simulink library "GaitPlayback"  (R2016b)
settings: Solver=VariableStepAuto  StartTime=0.0  StopTime=10.0  RelTol=1e-3
undefined symbols (not defined in the file or in its folder): halfStepStandStartHip, halfStepStandStartKnee, halfStepStopFromStandHip, halfStepStopFromStandKnee, halfStepStopFromSwingHip, halfStepStopFromSwingKnee, halfStepSwingStartHip, halfStepSwingStartKnee, initializeSitDownHip, initializeSitDownKnee, initializeSlopeDownHip, initializeSlopeDownKnee, initializeSlopeUpHip, initializeSlopeUpKnee, initializeSofaDownHip, initializeSofaDownKnee, initializeSofaUpHip, initializeSofaUpKnee, initializeStairsDownHip, initializeStairsDownKnee, initializeStairsUpHip, initializeStairsUpKnee, initializeStandUpHip, initializeStandUpKnee, roughTerrainStepLeftHip, roughTerrainStepLeftKnee, roughTerrainStepRightHip, roughTerrainStepRightKnee, sitDownHip, sitDownKnee, slopeDownLeftHip, slopeDownLeftKnee, slopeDownRightHip, slopeDownRightKnee, slopeUpLeftHip, slopeUpLeftKnee, slopeUpRightHip, slopeUpRightKnee, sofaDownHip, sofaDownKnee, sofaUpHip, sofaUpKnee, stairsDownLeftHip, stairsDownLeftKnee, stairsDownRightHip, stairsDownRightKnee, stairsUpLeftHip, stairsUpLeftKnee, stairsUpRightHip, stairsUpRightKnee, standUpHip, standUpKnee, stepStandLegHip, stepStandLegKnee, stepSwingLegHip, stepSwingLegKnee
libraries: lookUpTotalGaitDynamics x20, GaitPlayback x7, lookUpGaitDynamics x4, VariousLibrary x1
settings Model: Creator=Nathan  LastModifiedBy=MARCH

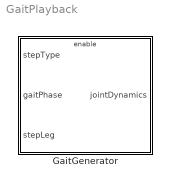
== system GaitPlayback ==
  GaitGenerator : Subsystem

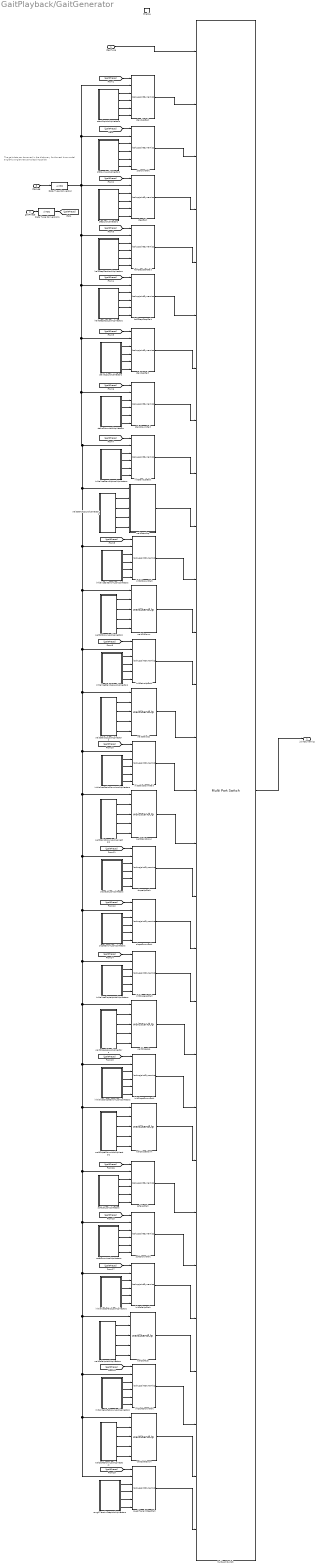
== system GaitPlayback/GaitGenerator ==
  note: The gait data can be saved in the dictionary for the real time model
      | angleHip
      | angleKnee
      | samplepoints/stride
  stepType : Inport
  gaitPhase : Inport  Port=2
  stepLeg : Inport  Port=3
  Enable : EnablePort
  Data Type Conversion : DataTypeConversion  OutDataTypeStr=uint32
  Data Type Conversion1 : DataTypeConversion  OutDataTypeStr=uint32  RndMeth=Nearest
  Multiport Switch : MultiPortSwitch  DataPortOrder=Specify indices  Inputs=4  DataPortIndices={StepType.STANDUP,StepType.SITDOWN,StepType.FULLSTEP,StepType.HALFSTEPSTART,StepType.HALFSTEPSTOP,StepType.STAIRSUPSTEP,StepType.STAIRSDOWNSTEP,StepType.INITIALIZESTANDUP,StepType.WAITSTANDUP,StepType.INITIALIZESITDOWN,StepType.WAITSITDOWN,StepType.INITIALIZESTAIRSUP,StepType.WAITSTAIRSUP,StepType.INITIALIZESTAIRSDOWN,StepType.WAITSTAIRSDOWN,StepType.SLOPEUPSTEP,StepType.SLOPEDOWNSTEP,StepType.INITIALIZESLOPEUP,StepType.WAITSLOPEUP,StepType.INITIALIZESLOPEDOWN,StepType.WAITSLOPEDOWN,StepType.SOFAUPSTEP,StepType.SOFADOWNSTEP,StepType.INITIALIZESOFAUP,StepType.WAITSOFAUP,StepType.INITIALIZESOFADOWN,StepType.WAITSOFADOWN,StepType.ROUGHTERRAINSTEP}  DiagnosticForDefault=None
  halfStepStartGait : lookUpTotalGaitDynamics/lookupJointDynamics
  halfStepStartLookUpVectors : Subsystem
  halfStepStopGait : lookUpTotalGaitDynamics/lookupJointDynamics
  halfStepStopLookUpVectors : Subsystem
  initSitDownGait : lookUpTotalGaitDynamics/lookupJointDynamics
  initSlopeDownGait : lookUpTotalGaitDynamics/lookupJointDynamics
  initSlopeUpGait : lookUpTotalGaitDynamics/lookupJointDynamics
  initSofaDownGait : lookUpTotalGaitDynamics/lookupJointDynamics
  initSofaUpGait : lookUpTotalGaitDynamics/lookupJointDynamics
  initStairsDownGait : lookUpTotalGaitDynamics/lookupJointDynamics
  initStairsUpGait : lookUpTotalGaitDynamics/lookupJointDynamics
  initStandUpGait : lookUpTotalGaitDynamics/lookupJointDynamics
  initializeSitDownLookUpVectors : Subsystem
  initializeSlopeDownLookUpVectors : Subsystem
  initializeSlopeUpLookUpVectors : Subsystem
  initializeSofaDownLookUpVectors : Subsystem
  initializeSofaUpLookUpVectors : Subsystem
  initializeStairsDownLookUpVectors : Subsystem
  initializeStairsUpLookUpVectors : Subsystem
  initializeStandUpLookUpVectors : Subsystem
  roughTerrainStepGait : lookUpTotalGaitDynamics/lookupJointDynamics
  roughTerrainStepLookUpVectors : Subsystem
  sitDownGait : lookUpTotalGaitDynamics/lookupJointDynamics
  sitDownLookUpVectors : Subsystem
  slopeDownGait : lookUpTotalGaitDynamics/lookupJointDynamics
  slopeDownLookUpVectors : Subsystem
  slopeUpGait : lookUpTotalGaitDynamics/lookupJointDynamics
  slopeUpLookUpVectors : Subsystem
  sofaDownGait : lookUpTotalGaitDynamics/lookupJointDynamics
  sofaDownLookUpVectors : Subsystem
  sofaUpGait : lookUpTotalGaitDynamics/lookupJointDynamics
  sofaUpLookUpVectors : Subsystem
  stairsDownGait : lookUpTotalGaitDynamics/lookupJointDynamics
  stairsDownLookUpVectors : Subsystem
  stairsUpGait : lookUpTotalGaitDynamics/lookupJointDynamics
  stairsUpLookUpVectors : Subsystem
  standUpGait : lookUpTotalGaitDynamics/lookupJointDynamics
  standUpLookUpVectors : Subsystem
  stepGait : lookUpTotalGaitDynamics/lookupJointDynamics
  stepLookUpVectors : Subsystem
  waitSitDown : GaitPlayback/GaitGenerator/waitStandUp
  waitSitDownLookUpVectors : Subsystem
  waitSlopeDown : GaitPlayback/GaitGenerator/waitStandUp
  waitSlopeDownLookUpVectors : Subsystem
  waitSlopeUp : GaitPlayback/GaitGenerator/waitStandUp
  waitSlopeUpLookUpVectors : Subsystem
  waitSofaDown : GaitPlayback/GaitGenerator/waitStandUp
  waitSofaDownLookUpVectors : Subsystem
  waitSofaUp : GaitPlayback/GaitGenerator/waitStandUp
  waitSofaUpLookUpVectors : Subsystem
  waitStairsDown : GaitPlayback/GaitGenerator/waitStandUp
  waitStairsDownLookUpVectors : Subsystem
  waitStairsUp : GaitPlayback/GaitGenerator/waitStandUp
  waitStairsUpLookUpVectors : Subsystem
  waitStandUp : Subsystem
  waitStandUpLookUpVectors : Subsystem
  jointDynamics : Outport  OutDataTypeStr=Bus: JointDynamics
  wires:
  stairsUpGait/1 -> Multiport Switch/7
  stairsDownGait/1 -> Multiport Switch/8
  stairsDownLookUpVectors/4(standLegKnee) -> stairsDownGait/6
  stairsDownLookUpVectors/3(standLegHip) -> stairsDownGait/5
  stairsDownLookUpVectors/2(swingLegKnee) -> stairsDownGait/4
  stairsDownLookUpVectors/1(swingLegHip) -> stairsDownGait/3
  [gaitPhase] -> stairsDownGait/1
  stairsUpLookUpVectors/4(standLegKnee) -> stairsUpGait/6
  stairsUpLookUpVectors/3(standLegHip) -> stairsUpGait/5
  stairsUpLookUpVectors/2(swingLegKnee) -> stairsUpGait/4
  stairsUpLookUpVectors/1(swingLegHip) -> stairsUpGait/3
  [gaitPhase] -> stairsUpGait/1
  standUpLookUpVectors/4(standLegKnee) -> standUpGait/6
  standUpLookUpVectors/3(standLegHip) -> standUpGait/5
  standUpLookUpVectors/2(swingLegKnee) -> standUpGait/4
  standUpLookUpVectors/1(swingLegHip) -> standUpGait/3
  gaitPhase/1 -> Data Type Conversion1/1
  Data Type Conversion1/1 -> [gaitPhase]
  [gaitPhase] -> halfStepStopGait/1
  halfStepStopLookUpVectors/4(standLegKnee) -> halfStepStopGait/6
  halfStepStopLookUpVectors/3(standLegHip) -> halfStepStopGait/5
  halfStepStopLookUpVectors/2(swingLegKnee) -> halfStepStopGait/4
  halfStepStopLookUpVectors/1(swingLegHip) -> halfStepStopGait/3
  halfStepStartLookUpVectors/4(standLegKnee) -> halfStepStartGait/6
  halfStepStartLookUpVectors/3(standLegHip) -> halfStepStartGait/5
  halfStepStartLookUpVectors/2(swingLegKnee) -> halfStepStartGait/4
  halfStepStartLookUpVectors/1(swingLegHip) -> halfStepStartGait/3
  sitDownLookUpVectors/1(swingLegHip) -> sitDownGait/3
  sitDownLookUpVectors/2(swingLegKnee) -> sitDownGait/4
  stepLookUpVectors/4(standLegKnee) -> stepGait/6
  [gaitPhase] -> halfStepStartGait/1
  [gaitPhase] -> stepGait/1
  [gaitPhase] -> standUpGait/1
  [gaitPhase] -> sitDownGait/1
  sitDownLookUpVectors/4(standLegKnee) -> sitDownGait/6
  sitDownLookUpVectors/3(standLegHip) -> sitDownGait/5
  stepLookUpVectors/3(standLegHip) -> stepGait/5
  stepLookUpVectors/2(swingLegKnee) -> stepGait/4
  stepLookUpVectors/1(swingLegHip) -> stepGait/3
  halfStepStopGait/1 -> Multiport Switch/6
  halfStepStartGait/1 -> Multiport Switch/5
  stepGait/1 -> Multiport Switch/4
  Multiport Switch/1 -> jointDynamics/1
  standUpGait/1 -> Multiport Switch/2
  stepType/1 -> Multiport Switch/1
  sitDownGait/1 -> Multiport Switch/3
  stepLeg/1 -> Data Type Conversion/1
  initStandUpGait/1 -> Multiport Switch/9
  initializeStandUpLookUpVectors/3(standLegHip) -> initStandUpGait/5
  initializeStandUpLookUpVectors/2(swingLegKnee) -> initStandUpGait/4
  initializeStandUpLookUpVectors/1(swingLegHip) -> initStandUpGait/3
  [gaitPhase] -> initStandUpGait/1
  initializeStandUpLookUpVectors/4(standLegKnee) -> initStandUpGait/6
  waitStandUpLookUpVectors/3(standLegHip) -> waitStandUp/4(standLegHip)
  waitStandUpLookUpVectors/2(swingLegKnee) -> waitStandUp/3(swingLegKnee)
  waitStandUpLookUpVectors/1(swingLegHip) -> waitStandUp/2(swingLegHip)
  waitStandUp/1(jointDynamics1) -> Multiport Switch/10
  waitStandUpLookUpVectors/4(standLegKnee) -> waitStandUp/5(standLegKnee)
  waitSitDownLookUpVectors/3(standLegHip) -> waitSitDown/4
  waitSitDownLookUpVectors/2(swingLegKnee) -> waitSitDown/3
  waitSitDownLookUpVectors/1(swingLegHip) -> waitSitDown/2
  waitSitDown/1 -> Multiport Switch/12
  waitSitDownLookUpVectors/4(standLegKnee) -> waitSitDown/5
  initSitDownGait/1 -> Multiport Switch/11
  initializeSitDownLookUpVectors/3(standLegHip) -> initSitDownGait/5
  initializeSitDownLookUpVectors/2(swingLegKnee) -> initSitDownGait/4
  initializeSitDownLookUpVectors/1(swingLegHip) -> initSitDownGait/3
  [gaitPhase] -> initSitDownGait/1
  initializeSitDownLookUpVectors/4(standLegKnee) -> initSitDownGait/6
  waitStairsUpLookUpVectors/3(standLegHip) -> waitStairsUp/4
  waitStairsUpLookUpVectors/2(swingLegKnee) -> waitStairsUp/3
  waitStairsUpLookUpVectors/1(swingLegHip) -> waitStairsUp/2
  waitStairsUpLookUpVectors/4(standLegKnee) -> waitStairsUp/5
  initializeStairsUpLookUpVectors/3(standLegHip) -> initStairsUpGait/5
  initializeStairsUpLookUpVectors/4(standLegKnee) -> initStairsUpGait/6
  initializeStairsUpLookUpVectors/2(swingLegKnee) -> initStairsUpGait/4
  initializeStairsUpLookUpVectors/1(swingLegHip) -> initStairsUpGait/3
  [gaitPhase] -> initStairsUpGait/1
  waitStairsDownLookUpVectors/3(standLegHip) -> waitStairsDown/4
  waitStairsDownLookUpVectors/2(swingLegKnee) -> waitStairsDown/3
  waitStairsDownLookUpVectors/1(swingLegHip) -> waitStairsDown/2
  waitStairsDownLookUpVectors/4(standLegKnee) -> waitStairsDown/5
  initializeStairsDownLookUpVectors/3(standLegHip) -> initStairsDownGait/5
  initializeStairsDownLookUpVectors/4(standLegKnee) -> initStairsDownGait/6
  initializeStairsDownLookUpVectors/2(swingLegKnee) -> initStairsDownGait/4
  initializeStairsDownLookUpVectors/1(swingLegHip) -> initStairsDownGait/3
  [gaitPhase] -> initStairsDownGait/1
  waitStairsDown/1 -> Multiport Switch/16
  initStairsDownGait/1 -> Multiport Switch/15
  waitStairsUp/1 -> Multiport Switch/14
  initStairsUpGait/1 -> Multiport Switch/13
  slopeUpGait/1 -> Multiport Switch/17
  slopeDownGait/1 -> Multiport Switch/18
  slopeDownLookUpVectors/4(standLegKnee) -> slopeDownGait/6
  slopeDownLookUpVectors/3(standLegHip) -> slopeDownGait/5
  slopeDownLookUpVectors/2(swingLegKnee) -> slopeDownGait/4
  slopeDownLookUpVectors/1(swingLegHip) -> slopeDownGait/3
  [gaitPhase] -> slopeDownGait/1
  slopeUpLookUpVectors/4(standLegKnee) -> slopeUpGait/6
  slopeUpLookUpVectors/3(standLegHip) -> slopeUpGait/5
  slopeUpLookUpVectors/2(swingLegKnee) -> slopeUpGait/4
  slopeUpLookUpVectors/1(swingLegHip) -> slopeUpGait/3
  [gaitPhase] -> slopeUpGait/1
  waitSlopeUpLookUpVectors/3(standLegHip) -> waitSlopeUp/4
  waitSlopeUpLookUpVectors/2(swingLegKnee) -> waitSlopeUp/3
  waitSlopeUpLookUpVectors/1(swingLegHip) -> waitSlopeUp/2
  waitSlopeUpLookUpVectors/4(standLegKnee) -> waitSlopeUp/5
  initializeSlopeUpLookUpVectors/3(standLegHip) -> initSlopeUpGait/5
  initializeSlopeUpLookUpVectors/4(standLegKnee) -> initSlopeUpGait/6
  initializeSlopeUpLookUpVectors/2(swingLegKnee) -> initSlopeUpGait/4
  initializeSlopeUpLookUpVectors/1(swingLegHip) -> initSlopeUpGait/3
  [gaitPhase] -> initSlopeUpGait/1
  waitSlopeDownLookUpVectors/3(standLegHip) -> waitSlopeDown/4
  waitSlopeDownLookUpVectors/2(swingLegKnee) -> waitSlopeDown/3
  waitSlopeDownLookUpVectors/1(swingLegHip) -> waitSlopeDown/2
  waitSlopeDownLookUpVectors/4(standLegKnee) -> waitSlopeDown/5
  initializeSlopeDownLookUpVectors/3(standLegHip) -> initSlopeDownGait/5
  initializeSlopeDownLookUpVectors/4(standLegKnee) -> initSlopeDownGait/6
  initializeSlopeDownLookUpVectors/2(swingLegKnee) -> initSlopeDownGait/4
  initializeSlopeDownLookUpVectors/1(swingLegHip) -> initSlopeDownGait/3
  [gaitPhase] -> initSlopeDownGait/1
  waitSlopeDown/1 -> Multiport Switch/22
  initSlopeDownGait/1 -> Multiport Switch/21
  waitSlopeUp/1 -> Multiport Switch/20
  initSlopeUpGait/1 -> Multiport Switch/19
  sofaUpLookUpVectors/4(standLegKnee) -> sofaUpGait/6
  sofaUpLookUpVectors/3(standLegHip) -> sofaUpGait/5
  sofaUpLookUpVectors/2(swingLegKnee) -> sofaUpGait/4
  sofaUpLookUpVectors/1(swingLegHip) -> sofaUpGait/3
  sofaDownLookUpVectors/1(swingLegHip) -> sofaDownGait/3
  [gaitPhase] -> sofaUpGait/1
  [gaitPhase] -> sofaDownGait/1
  sofaUpGait/1 -> Multiport Switch/23
  sofaDownGait/1 -> Multiport Switch/24
  initSofaUpGait/1 -> Multiport Switch/25
  initializeSofaUpLookUpVectors/3(standLegHip) -> initSofaUpGait/5
  initializeSofaUpLookUpVectors/2(swingLegKnee) -> initSofaUpGait/4
  initializeSofaUpLookUpVectors/1(swingLegHip) -> initSofaUpGait/3
  [gaitPhase] -> initSofaUpGait/1
  initializeSofaUpLookUpVectors/4(standLegKnee) -> initSofaUpGait/6
  waitSofaUpLookUpVectors/3(standLegHip) -> waitSofaUp/4
  waitSofaUpLookUpVectors/2(swingLegKnee) -> waitSofaUp/3
  waitSofaUpLookUpVectors/1(swingLegHip) -> waitSofaUp/2
  waitSofaUp/1 -> Multiport Switch/26
  waitSofaUpLookUpVectors/4(standLegKnee) -> waitSofaUp/5
  waitSofaDownLookUpVectors/3(standLegHip) -> waitSofaDown/4
  waitSofaDownLookUpVectors/2(swingLegKnee) -> waitSofaDown/3
  waitSofaDownLookUpVectors/1(swingLegHip) -> waitSofaDown/2
  waitSofaDown/1 -> Multiport Switch/28
  waitSofaDownLookUpVectors/4(standLegKnee) -> waitSofaDown/5
  initSofaDownGait/1 -> Multiport Switch/27
  initializeSofaDownLookUpVectors/3(standLegHip) -> initSofaDownGait/5
  initializeSofaDownLookUpVectors/2(swingLegKnee) -> initSofaDownGait/4
  initializeSofaDownLookUpVectors/1(swingLegHip) -> initSofaDownGait/3
  [gaitPhase] -> initSofaDownGait/1
  initializeSofaDownLookUpVectors/4(standLegKnee) -> initSofaDownGait/6
  sofaDownLookUpVectors/2(swingLegKnee) -> sofaDownGait/4
  sofaDownLookUpVectors/3(standLegHip) -> sofaDownGait/5
  sofaDownLookUpVectors/4(standLegKnee) -> sofaDownGait/6
  roughTerrainStepLookUpVectors/4(standLegKnee) -> roughTerrainStepGait/6
  roughTerrainStepLookUpVectors/3(standLegHip) -> roughTerrainStepGait/5
  roughTerrainStepLookUpVectors/2(swingLegKnee) -> roughTerrainStepGait/4
  roughTerrainStepLookUpVectors/1(swingLegHip) -> roughTerrainStepGait/3
  [gaitPhase] -> roughTerrainStepGait/1
  roughTerrainStepGait/1 -> Multiport Switch/29
  Data Type Conversion/1 -> standUpGait/2, sitDownGait/2, stairsDownGait/2, initSitDownGait/2, initStairsDownGait/2, initSlopeUpGait/2, waitSlopeUp/1, initSlopeDownGait/2, roughTerrainStepGait/2, waitSofaDown/1, initSofaDownGait/2, waitSofaUp/1, initSofaUpGait/2, sofaDownGait/2, sofaUpGait/2, waitSlopeDown/1, slopeDownGait/2, slopeUpGait/2, waitStairsDown/1, waitStairsUp/1, initStairsUpGait/2, waitSitDown/1, waitStandUp/1(stepLeg), initStandUpGait/2, stairsUpGait/2, halfStepStopGait/2, halfStepStartGait/2, stepGait/2

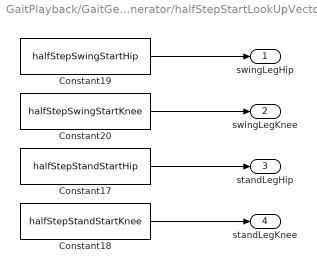
== system GaitPlayback/GaitGenerator/halfStepStartLookUpVectors ==
  Constant17 : Constant  Value=halfStepStandStartHip
  Constant18 : Constant  Value=halfStepStandStartKnee
  Constant19 : Constant  Value=halfStepSwingStartHip
  Constant20 : Constant  Value=halfStepSwingStartKnee
  swingLegHip : Outport
  swingLegKnee : Outport  Port=2
  standLegHip : Outport  Port=3
  standLegKnee : Outport  Port=4
  wires:
  Constant18/1 -> standLegKnee/1
  Constant17/1 -> standLegHip/1
  Constant19/1 -> swingLegHip/1
  Constant20/1 -> swingLegKnee/1

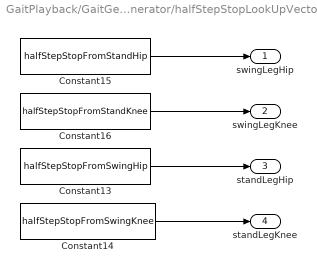
== system GaitPlayback/GaitGenerator/halfStepStopLookUpVectors ==
  Constant13 : Constant  Value=halfStepStopFromSwingHip
  Constant14 : Constant  Value=halfStepStopFromSwingKnee
  Constant15 : Constant  Value=halfStepStopFromStandHip
  Constant16 : Constant  Value=halfStepStopFromStandKnee
  swingLegHip : Outport
  swingLegKnee : Outport  Port=2
  standLegHip : Outport  Port=3
  standLegKnee : Outport  Port=4
  wires:
  Constant14/1 -> standLegKnee/1
  Constant13/1 -> standLegHip/1
  Constant15/1 -> swingLegHip/1
  Constant16/1 -> swingLegKnee/1

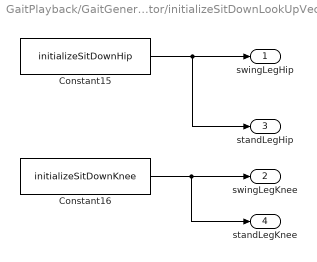
== system GaitPlayback/GaitGenerator/initializeSitDownLookUpVectors ==
  Constant15 : Constant  Value=initializeSitDownHip
  Constant16 : Constant  Value=initializeSitDownKnee
  swingLegHip : Outport
  swingLegKnee : Outport  Port=2
  standLegHip : Outport  Port=3
  standLegKnee : Outport  Port=4
  wires:
  Constant16/1 -> standLegKnee/1, swingLegKnee/1
  Constant15/1 -> standLegHip/1, swingLegHip/1

== system GaitPlayback/GaitGenerator/initializeSlopeDownLookUpVectors ==
  Constant15 : Constant  Value=initializeSlopeDownHip
  Constant16 : Constant  Value=initializeSlopeDownKnee
  swingLegHip : Outport
  swingLegKnee : Outport  Port=2
  standLegHip : Outport  Port=3
  standLegKnee : Outport  Port=4
  wires:
  Constant16/1 -> standLegKnee/1, swingLegKnee/1
  Constant15/1 -> standLegHip/1, swingLegHip/1

== system GaitPlayback/GaitGenerator/initializeSlopeUpLookUpVectors ==
  Constant15 : Constant  Value=initializeSlopeUpHip
  Constant16 : Constant  Value=initializeSlopeUpKnee
  swingLegHip : Outport
  swingLegKnee : Outport  Port=2
  standLegHip : Outport  Port=3
  standLegKnee : Outport  Port=4
  wires:
  Constant16/1 -> standLegKnee/1, swingLegKnee/1
  Constant15/1 -> standLegHip/1, swingLegHip/1

== system GaitPlayback/GaitGenerator/initializeSofaDownLookUpVectors ==
  Constant15 : Constant  Value=initializeSofaDownHip
  Constant16 : Constant  Value=initializeSofaDownKnee
  swingLegHip : Outport
  swingLegKnee : Outport  Port=2
  standLegHip : Outport  Port=3
  standLegKnee : Outport  Port=4
  wires:
  Constant16/1 -> standLegKnee/1, swingLegKnee/1
  Constant15/1 -> standLegHip/1, swingLegHip/1

== system GaitPlayback/GaitGenerator/initializeSofaUpLookUpVectors ==
  Constant15 : Constant  Value=initializeSofaUpHip
  Constant16 : Constant  Value=initializeSofaUpKnee
  swingLegHip : Outport
  swingLegKnee : Outport  Port=2
  standLegHip : Outport  Port=3
  standLegKnee : Outport  Port=4
  wires:
  Constant16/1 -> standLegKnee/1, swingLegKnee/1
  Constant15/1 -> standLegHip/1, swingLegHip/1

== system GaitPlayback/GaitGenerator/initializeStairsDownLookUpVectors ==
  Constant15 : Constant  Value=initializeStairsDownHip
  Constant16 : Constant  Value=initializeStairsDownKnee
  swingLegHip : Outport
  swingLegKnee : Outport  Port=2
  standLegHip : Outport  Port=3
  standLegKnee : Outport  Port=4
  wires:
  Constant16/1 -> standLegKnee/1, swingLegKnee/1
  Constant15/1 -> standLegHip/1, swingLegHip/1

== system GaitPlayback/GaitGenerator/initializeStairsUpLookUpVectors ==
  Constant15 : Constant  Value=initializeStairsUpHip
  Constant16 : Constant  Value=initializeStairsUpKnee
  swingLegHip : Outport
  swingLegKnee : Outport  Port=2
  standLegHip : Outport  Port=3
  standLegKnee : Outport  Port=4
  wires:
  Constant16/1 -> standLegKnee/1, swingLegKnee/1
  Constant15/1 -> standLegHip/1, swingLegHip/1

== system GaitPlayback/GaitGenerator/initializeStandUpLookUpVectors ==
  Constant15 : Constant  Value=initializeStandUpHip
  Constant16 : Constant  Value=initializeStandUpKnee
  swingLegHip : Outport
  swingLegKnee : Outport  Port=2
  standLegHip : Outport  Port=3
  standLegKnee : Outport  Port=4
  wires:
  Constant16/1 -> standLegKnee/1, swingLegKnee/1
  Constant15/1 -> standLegHip/1, swingLegHip/1

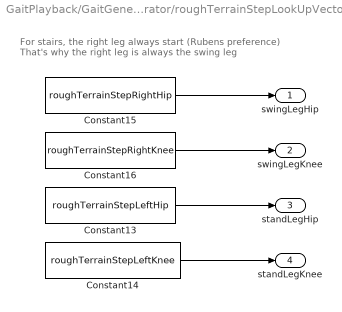
== system GaitPlayback/GaitGenerator/roughTerrainStepLookUpVectors ==
  note: For stairs, the right leg always start (Rubens preference)
      | That's why the right leg is always the swing leg
  Constant13 : Constant  Value=roughTerrainStepLeftHip
  Constant14 : Constant  Value=roughTerrainStepLeftKnee
  Constant15 : Constant  Value=roughTerrainStepRightHip
  Constant16 : Constant  Value=roughTerrainStepRightKnee
  swingLegHip : Outport
  swingLegKnee : Outport  Port=2
  standLegHip : Outport  Port=3
  standLegKnee : Outport  Port=4
  wires:
  Constant14/1 -> standLegKnee/1
  Constant13/1 -> standLegHip/1
  Constant15/1 -> swingLegHip/1
  Constant16/1 -> swingLegKnee/1

== system GaitPlayback/GaitGenerator/sitDownLookUpVectors ==
  Constant12 : Constant  Value=sitDownHip
  Constant7 : Constant  Value=sitDownKnee
  swingLegHip : Outport
  swingLegKnee : Outport  Port=2
  standLegHip : Outport  Port=3
  standLegKnee : Outport  Port=4
  wires:
  Constant12/1 -> swingLegHip/1, standLegHip/1
  Constant7/1 -> swingLegKnee/1, standLegKnee/1

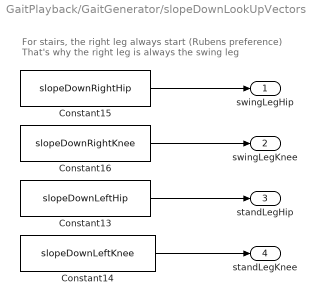
== system GaitPlayback/GaitGenerator/slopeDownLookUpVectors ==
  note: For stairs, the right leg always start (Rubens preference)
      | That's why the right leg is always the swing leg
  Constant13 : Constant  Value=slopeDownLeftHip
  Constant14 : Constant  Value=slopeDownLeftKnee
  Constant15 : Constant  Value=slopeDownRightHip
  Constant16 : Constant  Value=slopeDownRightKnee
  swingLegHip : Outport
  swingLegKnee : Outport  Port=2
  standLegHip : Outport  Port=3
  standLegKnee : Outport  Port=4
  wires:
  Constant14/1 -> standLegKnee/1
  Constant13/1 -> standLegHip/1
  Constant15/1 -> swingLegHip/1
  Constant16/1 -> swingLegKnee/1

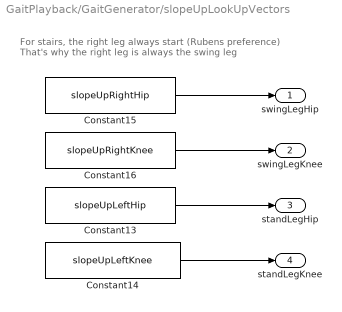
== system GaitPlayback/GaitGenerator/slopeUpLookUpVectors ==
  note: For stairs, the right leg always start (Rubens preference)
      | That's why the right leg is always the swing leg
  Constant13 : Constant  Value=slopeUpLeftHip
  Constant14 : Constant  Value=slopeUpLeftKnee
  Constant15 : Constant  Value=slopeUpRightHip
  Constant16 : Constant  Value=slopeUpRightKnee
  swingLegHip : Outport
  swingLegKnee : Outport  Port=2
  standLegHip : Outport  Port=3
  standLegKnee : Outport  Port=4
  wires:
  Constant14/1 -> standLegKnee/1
  Constant13/1 -> standLegHip/1
  Constant15/1 -> swingLegHip/1
  Constant16/1 -> swingLegKnee/1

== system GaitPlayback/GaitGenerator/sofaDownLookUpVectors ==
  Constant12 : Constant  Value=sofaDownHip
  Constant7 : Constant  Value=sofaDownKnee
  swingLegHip : Outport
  swingLegKnee : Outport  Port=2
  standLegHip : Outport  Port=3
  standLegKnee : Outport  Port=4
  wires:
  Constant12/1 -> swingLegHip/1, standLegHip/1
  Constant7/1 -> swingLegKnee/1, standLegKnee/1

== system GaitPlayback/GaitGenerator/sofaUpLookUpVectors ==
  standUpHip : Constant  Value=sofaUpHip
  standUpKnee : Constant  Value=sofaUpKnee
  swingLegHip : Outport
  swingLegKnee : Outport  Port=2
  standLegHip : Outport  Port=3
  standLegKnee : Outport  Port=4
  wires:
  standUpHip/1 -> swingLegHip/1, standLegHip/1
  standUpKnee/1 -> swingLegKnee/1, standLegKnee/1

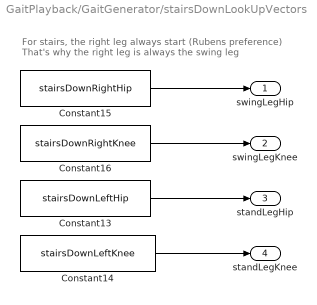
== system GaitPlayback/GaitGenerator/stairsDownLookUpVectors ==
  note: For stairs, the right leg always start (Rubens preference)
      | That's why the right leg is always the swing leg
  Constant13 : Constant  Value=stairsDownLeftHip
  Constant14 : Constant  Value=stairsDownLeftKnee
  Constant15 : Constant  Value=stairsDownRightHip
  Constant16 : Constant  Value=stairsDownRightKnee
  swingLegHip : Outport
  swingLegKnee : Outport  Port=2
  standLegHip : Outport  Port=3
  standLegKnee : Outport  Port=4
  wires:
  Constant14/1 -> standLegKnee/1
  Constant13/1 -> standLegHip/1
  Constant15/1 -> swingLegHip/1
  Constant16/1 -> swingLegKnee/1

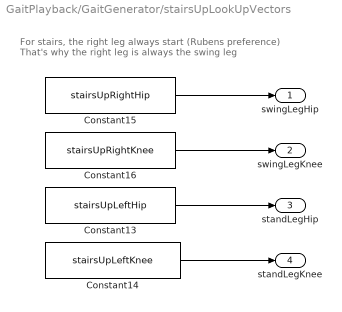
== system GaitPlayback/GaitGenerator/stairsUpLookUpVectors ==
  note: For stairs, the right leg always start (Rubens preference)
      | That's why the right leg is always the swing leg
  Constant13 : Constant  Value=stairsUpLeftHip
  Constant14 : Constant  Value=stairsUpLeftKnee
  Constant15 : Constant  Value=stairsUpRightHip
  Constant16 : Constant  Value=stairsUpRightKnee
  swingLegHip : Outport
  swingLegKnee : Outport  Port=2
  standLegHip : Outport  Port=3
  standLegKnee : Outport  Port=4
  wires:
  Constant14/1 -> standLegKnee/1
  Constant13/1 -> standLegHip/1
  Constant15/1 -> swingLegHip/1
  Constant16/1 -> swingLegKnee/1

== system GaitPlayback/GaitGenerator/standUpLookUpVectors ==
  standUpHip : Constant  Value=standUpHip
  standUpKnee : Constant  Value=standUpKnee
  swingLegHip : Outport
  swingLegKnee : Outport  Port=2
  standLegHip : Outport  Port=3
  standLegKnee : Outport  Port=4
  wires:
  standUpHip/1 -> swingLegHip/1, standLegHip/1
  standUpKnee/1 -> swingLegKnee/1, standLegKnee/1

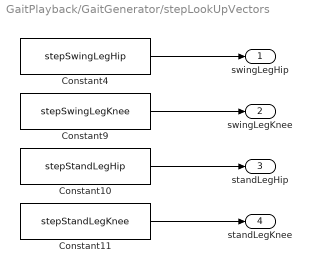
== system GaitPlayback/GaitGenerator/stepLookUpVectors ==
  Constant10 : Constant  Value=stepStandLegHip
  Constant11 : Constant  Value=stepStandLegKnee
  Constant4 : Constant  Value=stepSwingLegHip
  Constant9 : Constant  Value=stepSwingLegKnee
  swingLegHip : Outport
  swingLegKnee : Outport  Port=2
  standLegHip : Outport  Port=3
  standLegKnee : Outport  Port=4
  wires:
  Constant11/1 -> standLegKnee/1
  Constant10/1 -> standLegHip/1
  Constant4/1 -> swingLegHip/1
  Constant9/1 -> swingLegKnee/1

== system GaitPlayback/GaitGenerator/waitSitDownLookUpVectors ==
  Constant15 : Constant  Value=initializeSitDownHip(end)
  Constant2 : Constant  Value=initializeSitDownKnee(end)
  swingLegHip : Outport
  swingLegKnee : Outport  Port=2
  standLegHip : Outport  Port=3
  standLegKnee : Outport  Port=4
  wires:
  Constant2/1 -> swingLegKnee/1, standLegKnee/1
  Constant15/1 -> swingLegHip/1, standLegHip/1

== system GaitPlayback/GaitGenerator/waitSlopeDownLookUpVectors ==
  Constant15 : Constant  Value=initializeSlopeDownHip(end)
  Constant2 : Constant  Value=initializeSlopeDownKnee(end)
  swingLegHip : Outport
  swingLegKnee : Outport  Port=2
  standLegHip : Outport  Port=3
  standLegKnee : Outport  Port=4
  wires:
  Constant2/1 -> swingLegKnee/1, standLegKnee/1
  Constant15/1 -> swingLegHip/1, standLegHip/1

== system GaitPlayback/GaitGenerator/waitSlopeUpLookUpVectors ==
  Constant15 : Constant  Value=initializeSlopeUpHip(end)
  Constant2 : Constant  Value=initializeSlopeUpKnee(end)
  swingLegHip : Outport
  swingLegKnee : Outport  Port=2
  standLegHip : Outport  Port=3
  standLegKnee : Outport  Port=4
  wires:
  Constant2/1 -> swingLegKnee/1, standLegKnee/1
  Constant15/1 -> swingLegHip/1, standLegHip/1

== system GaitPlayback/GaitGenerator/waitSofaDownLookUpVectors ==
  Constant15 : Constant  Value=initializeSofaDownHip(end)
  Constant2 : Constant  Value=initializeSofaDownKnee(end)
  swingLegHip : Outport
  swingLegKnee : Outport  Port=2
  standLegHip : Outport  Port=3
  standLegKnee : Outport  Port=4
  wires:
  Constant2/1 -> swingLegKnee/1, standLegKnee/1
  Constant15/1 -> swingLegHip/1, standLegHip/1

== system GaitPlayback/GaitGenerator/waitSofaUpLookUpVectors ==
  Constant15 : Constant  Value=initializeSofaUpHip(end)
  Constant2 : Constant  Value=initializeSofaUpKnee(end)
  swingLegHip : Outport
  swingLegKnee : Outport  Port=2
  standLegHip : Outport  Port=3
  standLegKnee : Outport  Port=4
  wires:
  Constant15/1 -> swingLegHip/1, standLegHip/1
  Constant2/1 -> swingLegKnee/1, standLegKnee/1

== system GaitPlayback/GaitGenerator/waitStairsDownLookUpVectors ==
  Constant15 : Constant  Value=initializeStairsDownHip(end)
  Constant2 : Constant  Value=initializeStairsDownKnee(end)
  swingLegHip : Outport
  swingLegKnee : Outport  Port=2
  standLegHip : Outport  Port=3
  standLegKnee : Outport  Port=4
  wires:
  Constant2/1 -> swingLegKnee/1, standLegKnee/1
  Constant15/1 -> swingLegHip/1, standLegHip/1

== system GaitPlayback/GaitGenerator/waitStairsUpLookUpVectors ==
  Constant15 : Constant  Value=initializeStairsUpHip(end)
  Constant2 : Constant  Value=initializeStairsUpKnee(end)
  swingLegHip : Outport
  swingLegKnee : Outport  Port=2
  standLegHip : Outport  Port=3
  standLegKnee : Outport  Port=4
  wires:
  Constant2/1 -> swingLegKnee/1, standLegKnee/1
  Constant15/1 -> swingLegHip/1, standLegHip/1

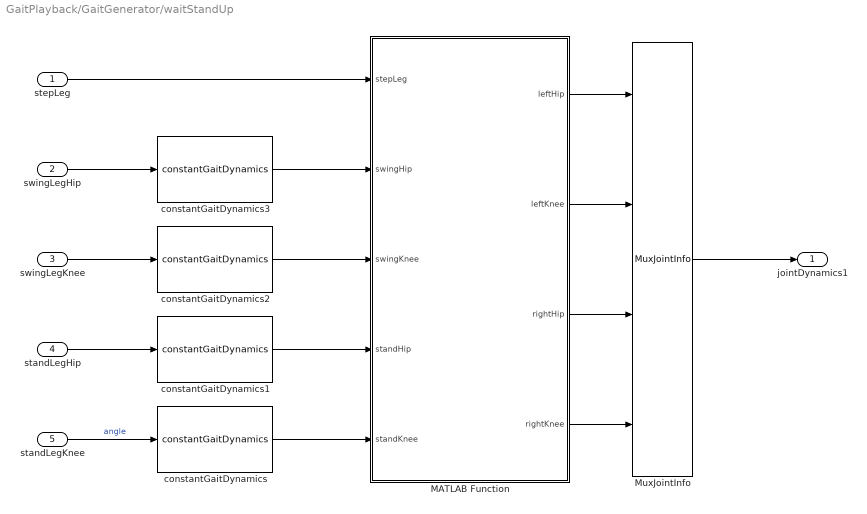
== system GaitPlayback/GaitGenerator/waitStandUp ==
  stepLeg : Inport
  swingLegHip : Inport  Port=2
  swingLegKnee : Inport  Port=3
  standLegHip : Inport  Port=4
  standLegKnee : Inport  Port=5
  MATLAB Function : MATLAB Function  TreatAsAtomicUnit=on
  MuxJointInfo : VariousLibrary/MuxJointInfo
  constantGaitDynamics{,1..3} (4 alike) : lookUpGaitDynamics/constantGaitDynamics
  jointDynamics1 : Outport  OutDataTypeStr=Bus: JointDynamics
  wires:
  MATLAB Function/4(rightKnee) -> MuxJointInfo/4
  MATLAB Function/3(rightHip) -> MuxJointInfo/3
  MATLAB Function/2(leftKnee) -> MuxJointInfo/2
  MATLAB Function/1(leftHip) -> MuxJointInfo/1
  constantGaitDynamics/1 -> MATLAB Function/5(standKnee)
  constantGaitDynamics1/1 -> MATLAB Function/4(standHip)
  constantGaitDynamics2/1 -> MATLAB Function/3(swingKnee)
  constantGaitDynamics3/1 -> MATLAB Function/2(swingHip)
  stepLeg/1 -> MATLAB Function/1(stepLeg)
  swingLegHip/1 -> constantGaitDynamics3/1
  swingLegKnee/1 -> constantGaitDynamics2/1
  standLegKnee/1 -> constantGaitDynamics/1  "angle"
  standLegHip/1 -> constantGaitDynamics1/1
  MuxJointInfo/1 -> jointDynamics1/1

== system GaitPlayback/GaitGenerator/waitStandUpLookUpVectors ==
  Constant15 : Constant  Value=initializeStandUpHip(end)
  Constant2 : Constant  Value=initializeStandUpKnee(end)
  swingLegHip : Outport
  swingLegKnee : Outport  Port=2
  standLegHip : Outport  Port=3
  standLegKnee : Outport  Port=4
  wires:
  Constant15/1 -> swingLegHip/1, standLegHip/1
  Constant2/1 -> swingLegKnee/1, standLegKnee/1

== matlab function GaitPlayback/GaitGenerator/waitStandUp/MATLAB Function ==
  data: stepLeg input; leftHip output Bus: JointDynamics; swingHip input Bus: JointDynamics; swingKnee input Bus: JointDynamics; standHip input Bus: JointDynamics; standKnee input Bus: JointDynamics; leftKnee output Bus: JointDynamics; rightHip output Bus: JointDynamics; rightKnee output Bus: JointDynamics
function [ leftHip, leftKnee, rightHip, rightKnee ] = routeSwingToLeg(stepLeg, swingHip, swingKnee, standHip, standKnee )
% wrapper for routeSwingToLeg
[ leftHip, leftKnee, rightHip, rightKnee ] = routeSwingToLeg(stepLeg, swingHip, swingKnee, standHip, standKnee );
end
